simulink model "NHR9410Model24k_2020b"  (R2020b)
settings: Solver=VariableStepAuto  StartTime=0.0  StopTime=1  FixedStep=0.001  RelTol=1e-3
libraries: simulink x85, fl_lib x46, powerlib_meascontrol x27, simulink_extras x24, nesl_utility x13, fl_ps_legacy_lib x3
(part 3 of 4)

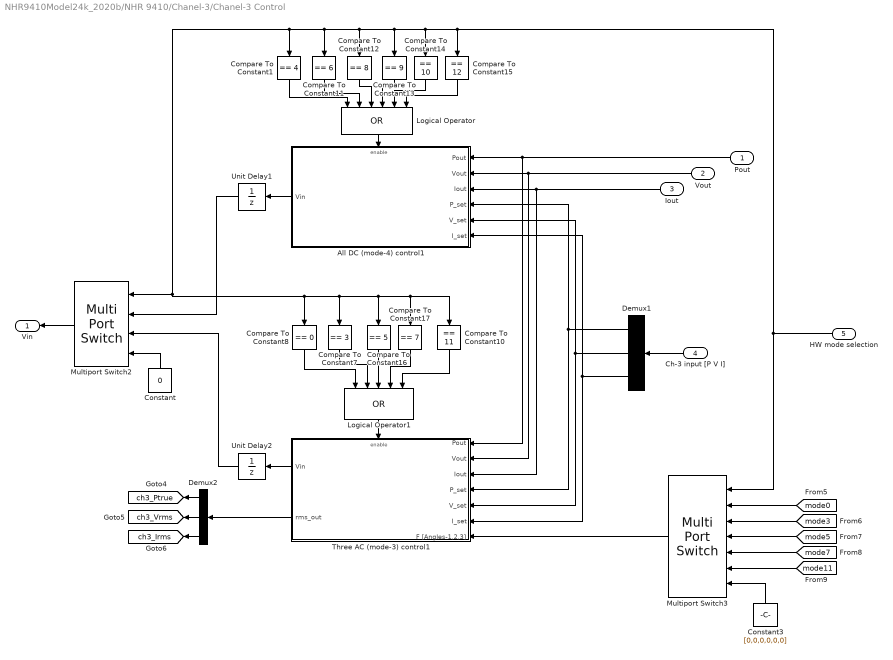
== system NHR9410Model24k_2020b/NHR 9410/Chanel-3/Chanel-3 Control ==
  Pout : Inport
  Vout : Inport  Port=2
  Iout : Inport  Port=3
  Ch-3 input [P V I] : Inport  Port=4
  HW mode selection : Inport  Port=5
  All DC (mode-4) control1 : Subsystem
      settings: MinAlgLoopOccurrences=on
  Compare To Constant1 : simulink/Logic and Bit Operations/Compare To Constant  relop===  const=4  OutDataTypeStr=boolean
  Compare To Constant10 : simulink/Logic and Bit Operations/Compare To Constant  relop===  const=11  OutDataTypeStr=boolean
  Compare To Constant11 : simulink/Logic and Bit Operations/Compare To Constant  relop===  const=6  OutDataTypeStr=boolean
  Compare To Constant12 : simulink/Logic and Bit Operations/Compare To Constant  relop===  const=8  OutDataTypeStr=boolean
  Compare To Constant13 : simulink/Logic and Bit Operations/Compare To Constant  relop===  const=9  OutDataTypeStr=boolean
  Compare To Constant14 : simulink/Logic and Bit Operations/Compare To Constant  relop===  const=10  OutDataTypeStr=boolean
  Compare To Constant15 : simulink/Logic and Bit Operations/Compare To Constant  relop===  const=12  OutDataTypeStr=boolean
  Compare To Constant16 : simulink/Logic and Bit Operations/Compare To Constant  relop===  const=5  OutDataTypeStr=boolean
  Compare To Constant17 : simulink/Logic and Bit Operations/Compare To Constant  relop===  const=7  OutDataTypeStr=boolean
  Compare To Constant7 : simulink/Logic and Bit Operations/Compare To Constant  relop===  const=3  OutDataTypeStr=boolean
  Compare To Constant8 : simulink/Logic and Bit Operations/Compare To Constant  relop===  const=0  OutDataTypeStr=boolean
  Constant : Constant  Value=0
  Constant3 : Constant  Value=[0,0,0,0,0,0]
  Demux1 : Demux  Outputs=3
  Demux2 : Demux  Outputs=3
  Logical Operator : Logic  Operator=OR  Inputs=6  AllPortsSameDT=off  OutDataTypeStr=boolean
  Logical Operator1 : Logic  Operator=OR  Inputs=5  AllPortsSameDT=off  OutDataTypeStr=boolean
  Multiport Switch2 : MultiPortSwitch  DataPortOrder=Specify indices  Inputs=13  DataPortIndices={[4,6,8,9,10,12],[0,3,5,7,11]}  DataPortForDefault=Additional data port  DiagnosticForDefault=None
  Multiport Switch3 : MultiPortSwitch  DataPortOrder=Specify indices  Inputs=13  DataPortIndices={0,3,5,7,11}  DataPortForDefault=Additional data port  DiagnosticForDefault=None
  Three AC (mode-3) control1 : Subsystem
      settings: MinAlgLoopOccurrences=on
  Unit Delay1 : UnitDelay  SampleTime=-1  HasFrameUpgradeWarning=on
  Unit Delay2 : UnitDelay  SampleTime=-1  HasFrameUpgradeWarning=on
  Vin : Outport  VectorParamsAs1DForOutWhenUnconnected=off
  tag scope: ch3_Irms=global, ch3_Ptrue=global, ch3_Vrms=global
  wires:
  Demux2/2 -> [ch3_Vrms]
  Demux2/3 -> [ch3_Irms]
  Demux2/1 -> [ch3_Ptrue]
  Multiport Switch3/1 -> Three AC (mode-3) control1/7(F [Angles-1,2,3])
  Compare To Constant17/1 -> Logical Operator1/4
  Iout/1 -> All DC (mode-4) control1/3(Iout), Three AC (mode-3) control1/3(Iout)
  Three AC (mode-3) control1/1(Vin) -> Unit Delay2/1
  Multiport Switch2/1 -> Vin/1
  [mode11] -> Multiport Switch3/6
  Logical Operator1/1 -> Three AC (mode-3) control1/Enable
  Demux1/1 -> All DC (mode-4) control1/4(P_set), Three AC (mode-3) control1/4(P_set)
  Compare To Constant10/1 -> Logical Operator1/5
  [mode0] -> Multiport Switch3/2
  Compare To Constant8/1 -> Logical Operator1/1
  Demux1/2 -> All DC (mode-4) control1/5(V_set), Three AC (mode-3) control1/5(V_set)
  Pout/1 -> All DC (mode-4) control1/1(Pout), Three AC (mode-3) control1/1(Pout)
  Demux1/3 -> All DC (mode-4) control1/6(I_set), Three AC (mode-3) control1/6(I_set)
  Vout/1 -> All DC (mode-4) control1/2(Vout), Three AC (mode-3) control1/2(Vout)
  [mode5] -> Multiport Switch3/4
  Ch-3 input [P V I]/1 -> Demux1/1
  [mode3] -> Multiport Switch3/3
  [mode7] -> Multiport Switch3/5
  Compare To Constant16/1 -> Logical Operator1/3
  All DC (mode-4) control1/1(Vin) -> Unit Delay1/1
  Constant3/1 -> Multiport Switch3/7
  Compare To Constant7/1 -> Logical Operator1/2
  Constant/1 -> Multiport Switch2/4
  Three AC (mode-3) control1/2(rms_out) -> Demux2/1
  Logical Operator/1 -> All DC (mode-4) control1/Enable
  Compare To Constant15/1 -> Logical Operator/6
  Compare To Constant14/1 -> Logical Operator/5
  Compare To Constant13/1 -> Logical Operator/4
  Compare To Constant1/1 -> Logical Operator/1
  Compare To Constant11/1 -> Logical Operator/2
  HW mode selection/1 -> Compare To Constant8/1, Compare To Constant10/1, Compare To Constant17/1, Compare To Constant16/1, Compare To Constant7/1, Multiport Switch2/1, Compare To Constant1/1, Compare To Constant11/1, Compare To Constant12/1, Compare To Constant13/1, Compare To Constant14/1, Compare To Constant15/1, Multiport Switch3/1
  Compare To Constant12/1 -> Logical Operator/3
  Unit Delay1/1 -> Multiport Switch2/2
  Unit Delay2/1 -> Multiport Switch2/3

== system NHR9410Model24k_2020b/NHR 9410 Safety Settings/Safety Ch-1/Trip signal generator (max) Sink Current ==
  signal_in : Inport
  Constant : Constant  Value=Simaxsnk1  VectorParams1D=off
  Constant1 : Constant  Value=0
  Relational Operator : RelationalOperator  OutDataTypeStr=boolean  RndMeth=Simplest
  trip signal gen : Subsystem
  signal_trip : Outport  VectorParamsAs1DForOutWhenUnconnected=off
  wires:
  signal_in/1 -> trip signal gen/1(signal in)
  trip signal gen/1(trip_out) -> signal_trip/1
  Constant/1 -> Relational Operator/1
  Constant1/1 -> Relational Operator/2
  Relational Operator/1 -> trip signal gen/Enable

== system NHR9410Model24k_2020b/NHR 9410 Safety Settings/Safety Ch-1/Trip signal generator (max) Sink Power ==
  signal_in : Inport
  Constant : Constant  Value=Spmaxsnk1  VectorParams1D=off
  Constant1 : Constant  Value=0
  Relational Operator : RelationalOperator  OutDataTypeStr=boolean  RndMeth=Simplest
  trip signal gen : Subsystem
  signal_trip : Outport  VectorParamsAs1DForOutWhenUnconnected=off
  wires:
  Relational Operator/1 -> trip signal gen/Enable
  Constant1/1 -> Relational Operator/2
  Constant/1 -> Relational Operator/1
  trip signal gen/1(trip_out) -> signal_trip/1
  signal_in/1 -> trip signal gen/1(signal in)

== system NHR9410Model24k_2020b/NHR 9410 Safety Settings/Safety Ch-1/Trip signal generator (max) Source Current ==
  signal_in : Inport
  Constant : Constant  Value=Simaxsrc1  VectorParams1D=off
  Constant1 : Constant  Value=0
  Relational Operator : RelationalOperator  OutDataTypeStr=boolean  RndMeth=Simplest
  trip signal gen : Subsystem
  signal_trip : Outport  VectorParamsAs1DForOutWhenUnconnected=off
  wires:
  Relational Operator/1 -> trip signal gen/Enable
  Constant1/1 -> Relational Operator/2
  Constant/1 -> Relational Operator/1
  trip signal gen/1(trip_out) -> signal_trip/1
  signal_in/1 -> trip signal gen/1(signal in)

== system NHR9410Model24k_2020b/NHR 9410 Safety Settings/Safety Ch-1/Trip signal generator (max) Source Power ==
  signal_in : Inport
  Constant : Constant  Value=Spmaxsrc1  VectorParams1D=off
  Constant1 : Constant  Value=0
  Relational Operator : RelationalOperator  OutDataTypeStr=boolean  RndMeth=Simplest
  trip signal gen : Subsystem
  signal_trip : Outport  VectorParamsAs1DForOutWhenUnconnected=off
  wires:
  signal_in/1 -> trip signal gen/1(signal in)
  trip signal gen/1(trip_out) -> signal_trip/1
  Constant/1 -> Relational Operator/1
  Constant1/1 -> Relational Operator/2
  Relational Operator/1 -> trip signal gen/Enable

== system NHR9410Model24k_2020b/NHR 9410 Safety Settings/Safety Ch-1/Trip signal generator (max) Voltage ==
  signal_in : Inport
  Constant : Constant  Value=Svmax1  VectorParams1D=off
  Constant1 : Constant  Value=0
  Relational Operator : RelationalOperator  OutDataTypeStr=boolean  RndMeth=Simplest
  trip signal gen : Subsystem
  signal_trip : Outport  VectorParamsAs1DForOutWhenUnconnected=off
  wires:
  signal_in/1 -> trip signal gen/1(signal in)
  trip signal gen/1(trip_out) -> signal_trip/1
  Constant/1 -> Relational Operator/1
  Constant1/1 -> Relational Operator/2
  Relational Operator/1 -> trip signal gen/Enable

== system NHR9410Model24k_2020b/NHR 9410 Safety Settings/Safety Ch-1/Trip signal generator (min) Voltage ==
  signal_in : Inport
  Constant : Constant  Value=Svmin1  VectorParams1D=off
  Constant1 : Constant  Value=0
  Relational Operator : RelationalOperator  OutDataTypeStr=boolean  RndMeth=Simplest
  trip signal gen : Subsystem
  signal_trip : Outport  VectorParamsAs1DForOutWhenUnconnected=off
  wires:
  Relational Operator/1 -> trip signal gen/Enable
  Constant1/1 -> Relational Operator/2
  Constant/1 -> Relational Operator/1
  trip signal gen/1(trip_out) -> signal_trip/1
  signal_in/1 -> trip signal gen/1(signal in)

== system NHR9410Model24k_2020b/NHR 9410 Safety Settings/Safety Ch-1/Trip signal generator (peak) Current ==
  signal_in : Inport
  peak_ctrl : Inport  Port=2
  Constant : Constant  Value=Ipeaken1  VectorParams1D=off
  Constant1 : Constant
  Logical Operator : Logic  AllPortsSameDT=off  OutDataTypeStr=boolean
  Relational Operator : RelationalOperator  Operator===  OutDataTypeStr=boolean  RndMeth=Simplest
  trip signal gen : Subsystem
  signal_trip : Outport  VectorParamsAs1DForOutWhenUnconnected=off
  wires:
  Constant1/1 -> Relational Operator/2
  Constant/1 -> Relational Operator/1
  signal_in/1 -> trip signal gen/1(signal in)
  trip signal gen/1(trip_out) -> signal_trip/1
  Relational Operator/1 -> Logical Operator/1
  Logical Operator/1 -> trip signal gen/Enable
  peak_ctrl/1 -> Logical Operator/2

== system NHR9410Model24k_2020b/NHR 9410 Safety Settings/Safety Ch-1/Trip signal generator (peak) Voltage ==
  signal_in : Inport
  peak_ctrl : Inport  Port=2
  Constant : Constant  Value=Vpeaken1  VectorParams1D=off
  Constant1 : Constant
  Logical Operator : Logic  AllPortsSameDT=off  OutDataTypeStr=boolean
  Relational Operator : RelationalOperator  Operator===  OutDataTypeStr=boolean  RndMeth=Simplest
  trip signal gen : Subsystem
  signal_trip : Outport  VectorParamsAs1DForOutWhenUnconnected=off
  wires:
  signal_in/1 -> trip signal gen/1(signal in)
  trip signal gen/1(trip_out) -> signal_trip/1
  Constant/1 -> Relational Operator/1
  Constant1/1 -> Relational Operator/2
  Relational Operator/1 -> Logical Operator/1
  Logical Operator/1 -> trip signal gen/Enable
  peak_ctrl/1 -> Logical Operator/2

== system NHR9410Model24k_2020b/NHR 9410 Safety Settings/Safety Ch-2/Trip signal generator (max) Sink Current ==
  signal_in : Inport
  Constant : Constant  Value=Simaxsnk2  VectorParams1D=off
  Constant1 : Constant  Value=0
  Relational Operator : RelationalOperator  OutDataTypeStr=boolean  RndMeth=Simplest
  trip signal gen : Subsystem
  signal_trip : Outport  VectorParamsAs1DForOutWhenUnconnected=off
  wires:
  Relational Operator/1 -> trip signal gen/Enable
  Constant1/1 -> Relational Operator/2
  Constant/1 -> Relational Operator/1
  trip signal gen/1(trip_out) -> signal_trip/1
  signal_in/1 -> trip signal gen/1(signal in)

== system NHR9410Model24k_2020b/NHR 9410 Safety Settings/Safety Ch-2/Trip signal generator (max) Sink Power ==
  signal_in : Inport
  Constant : Constant  Value=Spmaxsnk2  VectorParams1D=off
  Constant1 : Constant  Value=0
  Relational Operator : RelationalOperator  OutDataTypeStr=boolean  RndMeth=Simplest
  trip signal gen : Subsystem
  signal_trip : Outport  VectorParamsAs1DForOutWhenUnconnected=off
  wires:
  signal_in/1 -> trip signal gen/1(signal in)
  trip signal gen/1(trip_out) -> signal_trip/1
  Constant/1 -> Relational Operator/1
  Constant1/1 -> Relational Operator/2
  Relational Operator/1 -> trip signal gen/Enable

== system NHR9410Model24k_2020b/NHR 9410 Safety Settings/Safety Ch-2/Trip signal generator (max) Source Current ==
  signal_in : Inport
  Constant : Constant  Value=Simaxsrc2  VectorParams1D=off
  Constant1 : Constant  Value=0
  Relational Operator : RelationalOperator  OutDataTypeStr=boolean  RndMeth=Simplest
  trip signal gen : Subsystem
  signal_trip : Outport  VectorParamsAs1DForOutWhenUnconnected=off
  wires:
  signal_in/1 -> trip signal gen/1(signal in)
  trip signal gen/1(trip_out) -> signal_trip/1
  Constant/1 -> Relational Operator/1
  Constant1/1 -> Relational Operator/2
  Relational Operator/1 -> trip signal gen/Enable

== system NHR9410Model24k_2020b/NHR 9410 Safety Settings/Safety Ch-2/Trip signal generator (max) Source Power ==
  signal_in : Inport
  Constant : Constant  Value=Spmaxsrc2  VectorParams1D=off
  Constant1 : Constant  Value=0
  Relational Operator : RelationalOperator  OutDataTypeStr=boolean  RndMeth=Simplest
  trip signal gen : Subsystem
  signal_trip : Outport  VectorParamsAs1DForOutWhenUnconnected=off
  wires:
  Relational Operator/1 -> trip signal gen/Enable
  Constant1/1 -> Relational Operator/2
  Constant/1 -> Relational Operator/1
  trip signal gen/1(trip_out) -> signal_trip/1
  signal_in/1 -> trip signal gen/1(signal in)

== system NHR9410Model24k_2020b/NHR 9410 Safety Settings/Safety Ch-2/Trip signal generator (max) Voltage ==
  signal_in : Inport
  Constant : Constant  Value=Svmax2  VectorParams1D=off
  Constant1 : Constant  Value=0
  Relational Operator : RelationalOperator  OutDataTypeStr=boolean  RndMeth=Simplest
  trip signal gen : Subsystem
  signal_trip : Outport  VectorParamsAs1DForOutWhenUnconnected=off
  wires:
  Relational Operator/1 -> trip signal gen/Enable
  Constant1/1 -> Relational Operator/2
  Constant/1 -> Relational Operator/1
  trip signal gen/1(trip_out) -> signal_trip/1
  signal_in/1 -> trip signal gen/1(signal in)

== system NHR9410Model24k_2020b/NHR 9410 Safety Settings/Safety Ch-2/Trip signal generator (min) Voltage ==
  signal_in : Inport
  Constant : Constant  Value=Svmin2  VectorParams1D=off
  Constant1 : Constant  Value=0
  Relational Operator : RelationalOperator  OutDataTypeStr=boolean  RndMeth=Simplest
  trip signal gen : Subsystem
  signal_trip : Outport  VectorParamsAs1DForOutWhenUnconnected=off
  wires:
  signal_in/1 -> trip signal gen/1(signal in)
  trip signal gen/1(trip_out) -> signal_trip/1
  Constant/1 -> Relational Operator/1
  Constant1/1 -> Relational Operator/2
  Relational Operator/1 -> trip signal gen/Enable

== system NHR9410Model24k_2020b/NHR 9410 Safety Settings/Safety Ch-2/Trip signal generator (peak) Current ==
  signal_in : Inport
  peak_ctrl : Inport  Port=2
  Constant : Constant  Value=Ipeaken2  VectorParams1D=off
  Constant1 : Constant
  Logical Operator : Logic  AllPortsSameDT=off  OutDataTypeStr=boolean
  Relational Operator : RelationalOperator  Operator===  OutDataTypeStr=boolean  RndMeth=Simplest
  trip signal gen : Subsystem
  signal_trip : Outport  VectorParamsAs1DForOutWhenUnconnected=off
  wires:
  signal_in/1 -> trip signal gen/1(signal in)
  trip signal gen/1(trip_out) -> signal_trip/1
  Constant/1 -> Relational Operator/1
  Constant1/1 -> Relational Operator/2
  peak_ctrl/1 -> Logical Operator/2
  Relational Operator/1 -> Logical Operator/1
  Logical Operator/1 -> trip signal gen/Enable

== system NHR9410Model24k_2020b/NHR 9410 Safety Settings/Safety Ch-2/Trip signal generator (peak) Voltage ==
  signal_in : Inport
  peak_ctrl : Inport  Port=2
  Constant : Constant  Value=Vpeaken2  VectorParams1D=off
  Constant1 : Constant
  Logical Operator : Logic  AllPortsSameDT=off  OutDataTypeStr=boolean
  Relational Operator : RelationalOperator  Operator===  OutDataTypeStr=boolean  RndMeth=Simplest
  trip signal gen : Subsystem
  signal_trip : Outport  VectorParamsAs1DForOutWhenUnconnected=off
  wires:
  Constant1/1 -> Relational Operator/2
  Constant/1 -> Relational Operator/1
  trip signal gen/1(trip_out) -> signal_trip/1
  signal_in/1 -> trip signal gen/1(signal in)
  peak_ctrl/1 -> Logical Operator/2
  Logical Operator/1 -> trip signal gen/Enable
  Relational Operator/1 -> Logical Operator/1

== system NHR9410Model24k_2020b/NHR 9410 Safety Settings/Safety Ch-3/Trip signal generator (max) Sink Current ==
  signal_in : Inport
  Constant : Constant  Value=Simaxsnk3  VectorParams1D=off
  Constant1 : Constant  Value=0
  Relational Operator : RelationalOperator  OutDataTypeStr=boolean  RndMeth=Simplest
  trip signal gen : Subsystem
  signal_trip : Outport  VectorParamsAs1DForOutWhenUnconnected=off
  wires:
  signal_in/1 -> trip signal gen/1(signal in)
  trip signal gen/1(trip_out) -> signal_trip/1
  Constant/1 -> Relational Operator/1
  Constant1/1 -> Relational Operator/2
  Relational Operator/1 -> trip signal gen/Enable

== system NHR9410Model24k_2020b/NHR 9410 Safety Settings/Safety Ch-3/Trip signal generator (max) Sink Power ==
  signal_in : Inport
  Constant : Constant  Value=Spmaxsnk3  VectorParams1D=off
  Constant1 : Constant  Value=0
  Relational Operator : RelationalOperator  OutDataTypeStr=boolean  RndMeth=Simplest
  trip signal gen : Subsystem
  signal_trip : Outport  VectorParamsAs1DForOutWhenUnconnected=off
  wires:
  Relational Operator/1 -> trip signal gen/Enable
  Constant1/1 -> Relational Operator/2
  Constant/1 -> Relational Operator/1
  trip signal gen/1(trip_out) -> signal_trip/1
  signal_in/1 -> trip signal gen/1(signal in)

== system NHR9410Model24k_2020b/NHR 9410 Safety Settings/Safety Ch-3/Trip signal generator (max) Source Current ==
  signal_in : Inport
  Constant : Constant  Value=Simaxsrc3  VectorParams1D=off
  Constant1 : Constant  Value=0
  Relational Operator : RelationalOperator  OutDataTypeStr=boolean  RndMeth=Simplest
  trip signal gen : Subsystem
  signal_trip : Outport  VectorParamsAs1DForOutWhenUnconnected=off
  wires:
  Relational Operator/1 -> trip signal gen/Enable
  Constant1/1 -> Relational Operator/2
  Constant/1 -> Relational Operator/1
  trip signal gen/1(trip_out) -> signal_trip/1
  signal_in/1 -> trip signal gen/1(signal in)

== system NHR9410Model24k_2020b/NHR 9410 Safety Settings/Safety Ch-3/Trip signal generator (max) Source Power ==
  signal_in : Inport
  Constant : Constant  Value=Spmaxsrc3  VectorParams1D=off
  Constant1 : Constant  Value=0
  Relational Operator : RelationalOperator  OutDataTypeStr=boolean  RndMeth=Simplest
  trip signal gen : Subsystem
  signal_trip : Outport  VectorParamsAs1DForOutWhenUnconnected=off
  wires:
  signal_in/1 -> trip signal gen/1(signal in)
  trip signal gen/1(trip_out) -> signal_trip/1
  Constant/1 -> Relational Operator/1
  Constant1/1 -> Relational Operator/2
  Relational Operator/1 -> trip signal gen/Enable

== system NHR9410Model24k_2020b/NHR 9410 Safety Settings/Safety Ch-3/Trip signal generator (max) Voltage ==
  signal_in : Inport
  Constant : Constant  Value=Svmax3  VectorParams1D=off
  Constant1 : Constant  Value=0
  Relational Operator : RelationalOperator  OutDataTypeStr=boolean  RndMeth=Simplest
  trip signal gen : Subsystem
  signal_trip : Outport  VectorParamsAs1DForOutWhenUnconnected=off
  wires:
  signal_in/1 -> trip signal gen/1(signal in)
  trip signal gen/1(trip_out) -> signal_trip/1
  Constant/1 -> Relational Operator/1
  Constant1/1 -> Relational Operator/2
  Relational Operator/1 -> trip signal gen/Enable

== system NHR9410Model24k_2020b/NHR 9410 Safety Settings/Safety Ch-3/Trip signal generator (min) Voltage ==
  signal_in : Inport
  Constant : Constant  Value=Svmin3  VectorParams1D=off
  Constant1 : Constant  Value=0
  Relational Operator : RelationalOperator  OutDataTypeStr=boolean  RndMeth=Simplest
  trip signal gen : Subsystem
  signal_trip : Outport  VectorParamsAs1DForOutWhenUnconnected=off
  wires:
  Relational Operator/1 -> trip signal gen/Enable
  Constant1/1 -> Relational Operator/2
  Constant/1 -> Relational Operator/1
  trip signal gen/1(trip_out) -> signal_trip/1
  signal_in/1 -> trip signal gen/1(signal in)

== system NHR9410Model24k_2020b/NHR 9410 Safety Settings/Safety Ch-3/Trip signal generator (peak) Current ==
  signal_in : Inport
  peak_ctrl : Inport  Port=2
  Constant : Constant  Value=Ipeaken3  VectorParams1D=off
  Constant1 : Constant
  Logical Operator : Logic  AllPortsSameDT=off  OutDataTypeStr=boolean
  Relational Operator : RelationalOperator  Operator===  OutDataTypeStr=boolean  RndMeth=Simplest
  trip signal gen : Subsystem
  signal_trip : Outport  VectorParamsAs1DForOutWhenUnconnected=off
  wires:
  Constant1/1 -> Relational Operator/2
  Constant/1 -> Relational Operator/1
  trip signal gen/1(trip_out) -> signal_trip/1
  signal_in/1 -> trip signal gen/1(signal in)
  peak_ctrl/1 -> Logical Operator/2
  Logical Operator/1 -> trip signal gen/Enable
  Relational Operator/1 -> Logical Operator/1

== system NHR9410Model24k_2020b/NHR 9410 Safety Settings/Safety Ch-3/Trip signal generator (peak) Voltage ==
  signal_in : Inport
  peak_ctrl : Inport  Port=2
  Constant : Constant  Value=Vpeaken3  VectorParams1D=off
  Constant1 : Constant
  Logical Operator : Logic  AllPortsSameDT=off  OutDataTypeStr=boolean
  Relational Operator : RelationalOperator  Operator===  OutDataTypeStr=boolean  RndMeth=Simplest
  trip signal gen : Subsystem
  signal_trip : Outport  VectorParamsAs1DForOutWhenUnconnected=off
  wires:
  signal_in/1 -> trip signal gen/1(signal in)
  trip signal gen/1(trip_out) -> signal_trip/1
  Constant/1 -> Relational Operator/1
  Constant1/1 -> Relational Operator/2
  peak_ctrl/1 -> Logical Operator/2
  Logical Operator/1 -> trip signal gen/Enable
  Relational Operator/1 -> Logical Operator/1

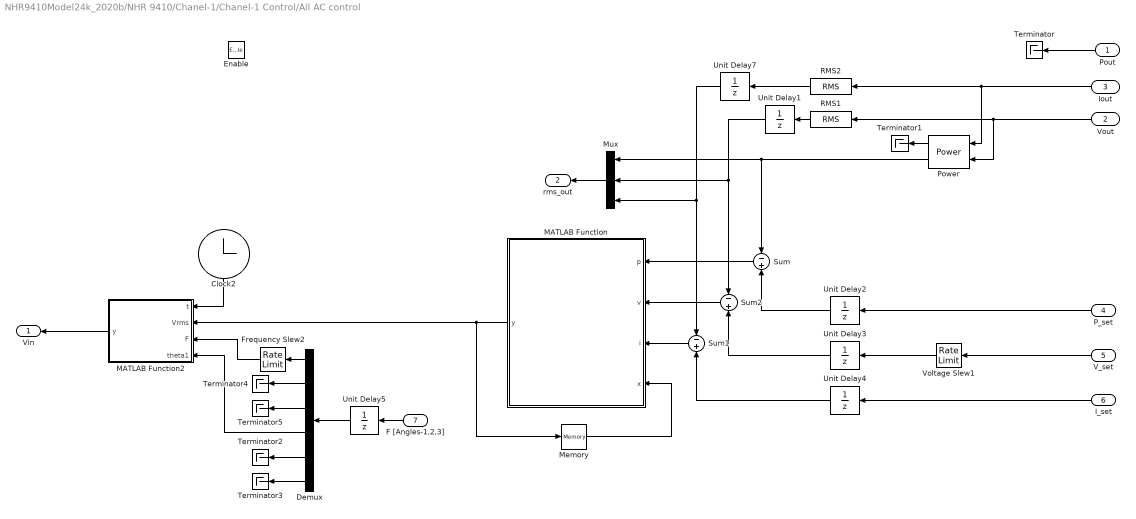
== system NHR9410Model24k_2020b/NHR 9410/Chanel-1/Chanel-1 Control/All AC control ==
  Pout : Inport
  Vout : Inport  Port=2
  Iout : Inport  Port=3
  P_set : Inport  Port=4
  V_set : Inport  Port=5
  I_set : Inport  Port=6
  F [Angles-1,2,3] : Inport  Port=7
  Enable : EnablePort
  Clock2 : Clock
  Demux : Demux  Outputs=6
  Frequency Slew2 : RateLimiter  RisingSlewLimit=FslewAC  FallingSlewLimit=-FslewAC  SampleTimeMode=inherited  LinearizeAsGain=off
  MATLAB Function : MATLAB Function  TreatAsAtomicUnit=on
  MATLAB Function2 : MATLAB Function  TreatAsAtomicUnit=on
  Memory : Memory
  Mux : Mux  Inputs=3
  Power : powerlib_meascontrol/Measurements/Power  Freq=60  Vinit=[0, 0]  Iinit=[0, 0]  Ts=0
  RMS1 : powerlib_meascontrol/Measurements/RMS  TrueRMS=on  Freq=60  RMSInit=0  Ts=0
  RMS2 : powerlib_meascontrol/Measurements/RMS  TrueRMS=on  Freq=60  RMSInit=0  Ts=0
  Sum : Sum  Inputs=-+
  Sum1 : Sum  Inputs=-+
  Sum2 : Sum  Inputs=-+
  Terminator{,1..5} (6 alike) : Terminator
  Unit Delay{1..5,7} (6 alike) : UnitDelay  SampleTime=-1  HasFrameUpgradeWarning=on
  Voltage Slew1 : RateLimiter  RisingSlewLimit=VslewAC  FallingSlewLimit=-VslewAC  SampleTimeMode=inherited  LinearizeAsGain=off
  Vin : Outport  VectorParamsAs1DForOutWhenUnconnected=off
  rms_out : Outport  Port=2  VectorParamsAs1DForOutWhenUnconnected=off
  wires:
  Voltage Slew1/1 -> Unit Delay3/1
  Frequency Slew2/1 -> MATLAB Function2/3(F)
  V_set/1 -> Voltage Slew1/1
  F [Angles-1,2,3]/1 -> Unit Delay5/1
  Demux/6 -> Terminator3/1
  Demux/3 -> Terminator5/1
  Mux/1 -> rms_out/1
  Power/1 -> Sum/1, Mux/1
  MATLAB Function2/1(y) -> Vin/1
  Clock2/1 -> MATLAB Function2/1(t)
  Memory/1 -> MATLAB Function/4(x)
  RMS2/1 -> Unit Delay7/1
  RMS1/1 -> Unit Delay1/1
  P_set/1 -> Unit Delay2/1
  I_set/1 -> Unit Delay4/1
  Sum1/1 -> MATLAB Function/3(i)
  Sum2/1 -> MATLAB Function/2(v)
  Sum/1 -> MATLAB Function/1(p)
  Power/2 -> Terminator1/1
  Pout/1 -> Terminator/1
  Iout/1 -> Power/2, RMS2/1
  MATLAB Function/1(y) -> Memory/1, MATLAB Function2/2(Vrms)
  Vout/1 -> Power/1, RMS1/1
  Demux/1 -> Frequency Slew2/1
  Demux/2 -> Terminator4/1
  Demux/5 -> Terminator2/1
  Demux/4 -> MATLAB Function2/4(theta1)
  Unit Delay7/1 -> Sum1/1, Mux/3
  Unit Delay1/1 -> Sum2/1, Mux/2
  Unit Delay2/1 -> Sum/2
  Unit Delay3/1 -> Sum2/2
  Unit Delay4/1 -> Sum1/2
  Unit Delay5/1 -> Demux/1

== system NHR9410Model24k_2020b/NHR 9410/Chanel-1/Chanel-1 Control/All DC control ==
  Pout : Inport
  Vout : Inport  Port=2
  Iout : Inport  Port=3
  P_set : Inport  Port=4
  V_set : Inport  Port=5
  I_set : Inport  Port=6
  Enable : EnablePort
  Current Slew : RateLimiter  RisingSlewLimit=IslewDC  FallingSlewLimit=-IslewDC  SampleTimeMode=inherited  LinearizeAsGain=off
  MATLAB Function : MATLAB Function  TreatAsAtomicUnit=on
  Memory : Memory
  Power Slew : RateLimiter  RisingSlewLimit=PslewDC  FallingSlewLimit=-PslewDC  SampleTimeMode=inherited  LinearizeAsGain=off
  Sum : Sum  Inputs=-+
  Sum1 : Sum  Inputs=-+
  Sum2 : Sum  Inputs=-+
  Unit Delay{,1..5} (6 alike) : UnitDelay  SampleTime=-1  HasFrameUpgradeWarning=on
  Voltage Slew : RateLimiter  RisingSlewLimit=VslewDC  FallingSlewLimit=-VslewDC  SampleTimeMode=inherited  LinearizeAsGain=off
  Vin : Outport  VectorParamsAs1DForOutWhenUnconnected=off
  wires:
  Power Slew/1 -> Unit Delay4/1
  Voltage Slew/1 -> Unit Delay3/1
  Current Slew/1 -> Unit Delay5/1
  I_set/1 -> Current Slew/1
  V_set/1 -> Voltage Slew/1
  P_set/1 -> Power Slew/1
  MATLAB Function/1(y) -> Memory/1, Vin/1
  Iout/1 -> Unit Delay/1
  Pout/1 -> Unit Delay2/1
  Sum/1 -> MATLAB Function/1(p)
  Sum1/1 -> MATLAB Function/3(i)
  Sum2/1 -> MATLAB Function/2(v)
  Memory/1 -> MATLAB Function/4(x)
  Unit Delay2/1 -> Sum/1
  Vout/1 -> Unit Delay1/1
  Unit Delay/1 -> Sum1/1
  Unit Delay1/1 -> Sum2/1
  Unit Delay4/1 -> Sum/2
  Unit Delay3/1 -> Sum2/2
  Unit Delay5/1 -> Sum1/2

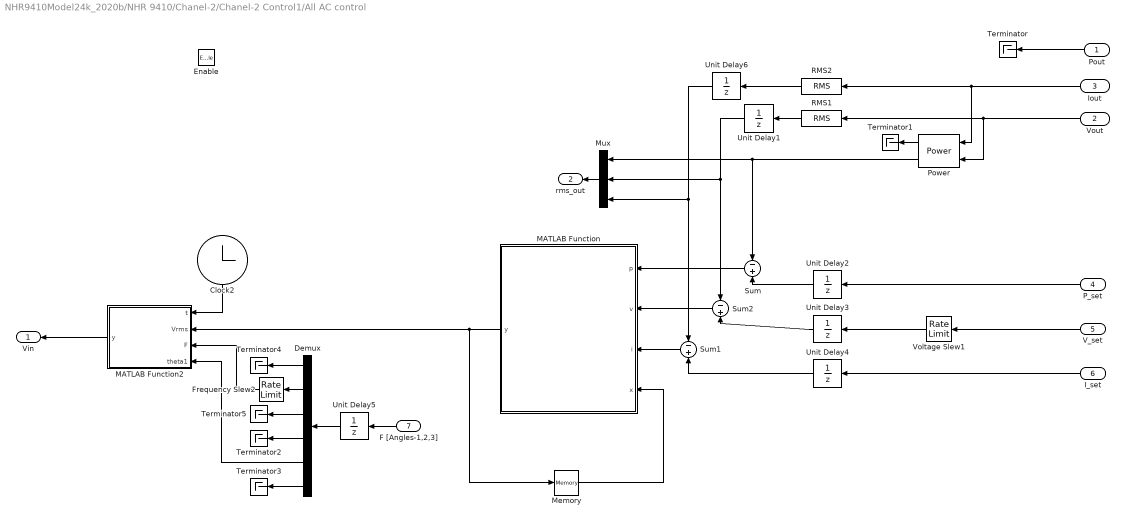
== system NHR9410Model24k_2020b/NHR 9410/Chanel-2/Chanel-2 Control1/All AC control ==
  Pout : Inport
  Vout : Inport  Port=2
  Iout : Inport  Port=3
  P_set : Inport  Port=4
  V_set : Inport  Port=5
  I_set : Inport  Port=6
  F [Angles-1,2,3] : Inport  Port=7
  Enable : EnablePort
  Clock2 : Clock
  Demux : Demux  Outputs=6
  Frequency Slew2 : RateLimiter  RisingSlewLimit=FslewAC  FallingSlewLimit=-FslewAC  SampleTimeMode=inherited  LinearizeAsGain=off
  MATLAB Function : MATLAB Function  TreatAsAtomicUnit=on
  MATLAB Function2 : MATLAB Function  TreatAsAtomicUnit=on
  Memory : Memory
  Mux : Mux  Inputs=3
  Power : powerlib_meascontrol/Measurements/Power  Freq=60  Vinit=[0, 0]  Iinit=[0, 0]  Ts=0
  RMS1 : powerlib_meascontrol/Measurements/RMS  TrueRMS=on  Freq=60  RMSInit=0  Ts=0
  RMS2 : powerlib_meascontrol/Measurements/RMS  TrueRMS=on  Freq=60  RMSInit=0  Ts=0
  Sum : Sum  Inputs=-+
  Sum1 : Sum  Inputs=-+
  Sum2 : Sum  Inputs=-+
  Terminator{,1..5} (6 alike) : Terminator
  Unit Delay{1..6} (6 alike) : UnitDelay  SampleTime=-1  HasFrameUpgradeWarning=on
  Voltage Slew1 : RateLimiter  RisingSlewLimit=VslewAC  FallingSlewLimit=-VslewAC  SampleTimeMode=inherited  LinearizeAsGain=off
  Vin : Outport  VectorParamsAs1DForOutWhenUnconnected=off
  rms_out : Outport  Port=2  VectorParamsAs1DForOutWhenUnconnected=off
  wires:
  Vout/1 -> RMS1/1, Power/1
  MATLAB Function/1(y) -> MATLAB Function2/2(Vrms), Memory/1
  Iout/1 -> RMS2/1, Power/2
  Pout/1 -> Terminator/1
  Power/2 -> Terminator1/1
  Sum/1 -> MATLAB Function/1(p)
  Sum2/1 -> MATLAB Function/2(v)
  Sum1/1 -> MATLAB Function/3(i)
  I_set/1 -> Unit Delay4/1
  P_set/1 -> Unit Delay2/1
  RMS1/1 -> Unit Delay1/1
  RMS2/1 -> Unit Delay6/1
  Memory/1 -> MATLAB Function/4(x)
  Clock2/1 -> MATLAB Function2/1(t)
  MATLAB Function2/1(y) -> Vin/1
  Power/1 -> Sum/1, Mux/1
  Mux/1 -> rms_out/1
  Demux/3 -> Terminator5/1
  Demux/6 -> Terminator3/1
  F [Angles-1,2,3]/1 -> Unit Delay5/1
  Demux/1 -> Terminator4/1
  Demux/4 -> Terminator2/1
  Demux/5 -> MATLAB Function2/4(theta1)
  V_set/1 -> Voltage Slew1/1
  Demux/2 -> Frequency Slew2/1
  Frequency Slew2/1 -> MATLAB Function2/3(F)
  Voltage Slew1/1 -> Unit Delay3/1
  Unit Delay6/1 -> Sum1/1, Mux/3
  Unit Delay1/1 -> Sum2/1, Mux/2
  Unit Delay2/1 -> Sum/2
  Unit Delay3/1 -> Sum2/2
  Unit Delay4/1 -> Sum1/2
  Unit Delay5/1 -> Demux/1

== system NHR9410Model24k_2020b/NHR 9410/Chanel-2/Chanel-2 Control1/All DC control ==
  Pout : Inport
  Vout : Inport  Port=2
  Iout : Inport  Port=3
  P_set : Inport  Port=4
  V_set : Inport  Port=5
  I_set : Inport  Port=6
  Enable : EnablePort
  Current Slew : RateLimiter  RisingSlewLimit=IslewDC  FallingSlewLimit=-IslewDC  SampleTimeMode=inherited  LinearizeAsGain=off
  MATLAB Function : MATLAB Function  TreatAsAtomicUnit=on
  Memory : Memory
  Power Slew : RateLimiter  RisingSlewLimit=PslewDC  FallingSlewLimit=-PslewDC  SampleTimeMode=inherited  LinearizeAsGain=off
  Sum : Sum  Inputs=-+
  Sum1 : Sum  Inputs=-+
  Sum2 : Sum  Inputs=-+
  Unit Delay{1..7} (7 alike) : UnitDelay  SampleTime=-1  HasFrameUpgradeWarning=on
  Voltage Slew : RateLimiter  RisingSlewLimit=VslewDC  FallingSlewLimit=-VslewDC  SampleTimeMode=inherited  LinearizeAsGain=off
  Vin : Outport  VectorParamsAs1DForOutWhenUnconnected=off
  wires:
  Memory/1 -> MATLAB Function/4(x)
  Sum2/1 -> MATLAB Function/2(v)
  Sum1/1 -> MATLAB Function/3(i)
  Sum/1 -> MATLAB Function/1(p)
  Pout/1 -> Unit Delay2/1
  Iout/1 -> Unit Delay3/1
  MATLAB Function/1(y) -> Unit Delay4/1
  P_set/1 -> Power Slew/1
  V_set/1 -> Voltage Slew/1
  I_set/1 -> Current Slew/1
  Current Slew/1 -> Unit Delay7/1
  Voltage Slew/1 -> Unit Delay6/1
  Power Slew/1 -> Unit Delay5/1
  Unit Delay2/1 -> Sum/1
  Vout/1 -> Unit Delay1/1
  Unit Delay3/1 -> Sum1/1
  Unit Delay4/1 -> Vin/1, Memory/1
  Unit Delay1/1 -> Sum2/1
  Unit Delay5/1 -> Sum/2
  Unit Delay6/1 -> Sum2/2
  Unit Delay7/1 -> Sum1/2

== system NHR9410Model24k_2020b/NHR 9410/Chanel-3/Chanel-3 Control/All DC (mode-4) control1 ==
  Pout : Inport
  Vout : Inport  Port=2
  Iout : Inport  Port=3
  P_set : Inport  Port=4
  V_set : Inport  Port=5
  I_set : Inport  Port=6
  Enable : EnablePort
  Current Slew : RateLimiter  RisingSlewLimit=IslewDC  FallingSlewLimit=-IslewDC  SampleTimeMode=inherited  LinearizeAsGain=off
  MATLAB Function : MATLAB Function  TreatAsAtomicUnit=on
  Memory : Memory
  Power Slew : RateLimiter  RisingSlewLimit=PslewDC  FallingSlewLimit=-PslewDC  SampleTimeMode=inherited  LinearizeAsGain=off
  Scope : Scope
  Sum : Sum  Inputs=-+
  Sum1 : Sum  Inputs=-+
  Sum2 : Sum  Inputs=-+
  Unit Delay{,1..5} (6 alike) : UnitDelay  SampleTime=-1  HasFrameUpgradeWarning=on
  Voltage Slew : RateLimiter  RisingSlewLimit=VslewDC  FallingSlewLimit=-VslewDC  SampleTimeMode=inherited  LinearizeAsGain=off
  Vin : Outport  VectorParamsAs1DForOutWhenUnconnected=off
  wires:
  Memory/1 -> MATLAB Function/4(x)
  Sum2/1 -> MATLAB Function/2(v)
  Sum1/1 -> MATLAB Function/3(i)
  Sum/1 -> MATLAB Function/1(p)
  MATLAB Function/1(y) -> Scope/1, Vin/1, Memory/1
  P_set/1 -> Power Slew/1
  V_set/1 -> Voltage Slew/1
  I_set/1 -> Current Slew/1
  Current Slew/1 -> Unit Delay2/1
  Voltage Slew/1 -> Unit Delay1/1
  Power Slew/1 -> Unit Delay3/1
  Pout/1 -> Unit Delay5/1
  Iout/1 -> Unit Delay4/1
  Vout/1 -> Unit Delay/1
  Unit Delay3/1 -> Sum/2
  Unit Delay1/1 -> Sum2/2
  Unit Delay2/1 -> Sum1/2
  Unit Delay4/1 -> Sum1/1
  Unit Delay/1 -> Sum2/1
  Unit Delay5/1 -> Sum/1

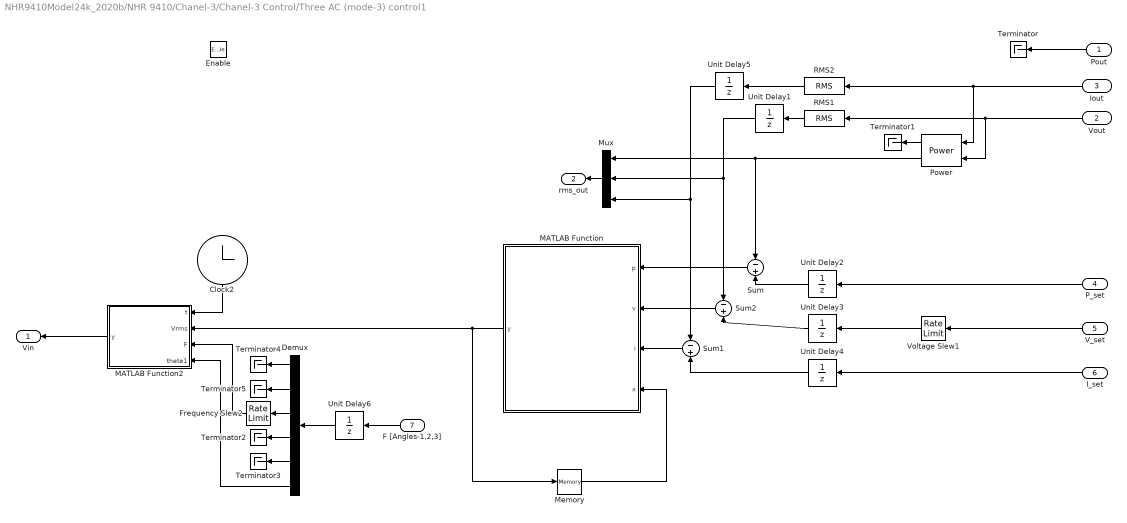
== system NHR9410Model24k_2020b/NHR 9410/Chanel-3/Chanel-3 Control/Three AC (mode-3) control1 ==
  Pout : Inport
  Vout : Inport  Port=2
  Iout : Inport  Port=3
  P_set : Inport  Port=4
  V_set : Inport  Port=5
  I_set : Inport  Port=6
  F [Angles-1,2,3] : Inport  Port=7
  Enable : EnablePort
  Clock2 : Clock
  Demux : Demux  Outputs=6
  Frequency Slew2 : RateLimiter  RisingSlewLimit=FslewAC  FallingSlewLimit=-FslewAC  SampleTimeMode=inherited  LinearizeAsGain=off
  MATLAB Function : MATLAB Function  TreatAsAtomicUnit=on
  MATLAB Function2 : MATLAB Function  TreatAsAtomicUnit=on
  Memory : Memory
  Mux : Mux  Inputs=3
  Power : powerlib_meascontrol/Measurements/Power  Freq=60  Vinit=[0, 0]  Iinit=[0, 0]  Ts=0
  RMS1 : powerlib_meascontrol/Measurements/RMS  TrueRMS=on  Freq=60  RMSInit=0  Ts=0
  RMS2 : powerlib_meascontrol/Measurements/RMS  TrueRMS=on  Freq=60  RMSInit=0  Ts=0
  Sum : Sum  Inputs=-+
  Sum1 : Sum  Inputs=-+
  Sum2 : Sum  Inputs=-+
  Terminator{,1..5} (6 alike) : Terminator
  Unit Delay{1..6} (6 alike) : UnitDelay  SampleTime=-1  HasFrameUpgradeWarning=on
  Voltage Slew1 : RateLimiter  RisingSlewLimit=VslewAC  FallingSlewLimit=-VslewAC  SampleTimeMode=inherited  LinearizeAsGain=off
  Vin : Outport  VectorParamsAs1DForOutWhenUnconnected=off
  rms_out : Outport  Port=2  VectorParamsAs1DForOutWhenUnconnected=off
  wires:
  Vout/1 -> RMS1/1, Power/1
  MATLAB Function/1(y) -> MATLAB Function2/2(Vrms), Memory/1
  Iout/1 -> RMS2/1, Power/2
  Pout/1 -> Terminator/1
  Power/2 -> Terminator1/1
  Sum/1 -> MATLAB Function/1(p)
  Sum2/1 -> MATLAB Function/2(v)
  Sum1/1 -> MATLAB Function/3(i)
  I_set/1 -> Unit Delay4/1
  P_set/1 -> Unit Delay2/1
  RMS1/1 -> Unit Delay1/1
  RMS2/1 -> Unit Delay5/1
  Memory/1 -> MATLAB Function/4(x)
  Clock2/1 -> MATLAB Function2/1(t)
  MATLAB Function2/1(y) -> Vin/1
  Power/1 -> Sum/1, Mux/1
  Mux/1 -> rms_out/1
  F [Angles-1,2,3]/1 -> Unit Delay6/1
  Demux/1 -> Terminator4/1
  Demux/4 -> Terminator2/1
  V_set/1 -> Voltage Slew1/1
  Demux/2 -> Terminator5/1
  Demux/5 -> Terminator3/1
  Demux/3 -> Frequency Slew2/1
  Demux/6 -> MATLAB Function2/4(theta1)
  Frequency Slew2/1 -> MATLAB Function2/3(F)
  Voltage Slew1/1 -> Unit Delay3/1
  Unit Delay5/1 -> Sum1/1, Mux/3
  Unit Delay1/1 -> Sum2/1, Mux/2
  Unit Delay2/1 -> Sum/2
  Unit Delay3/1 -> Sum2/2
  Unit Delay4/1 -> Sum1/2
  Unit Delay6/1 -> Demux/1

== system NHR9410Model24k_2020b/NHR 9410 Safety Settings/Safety Ch-1/Trip signal generator (max) Sink Current/trip signal gen ==
  signal in : Inport
  Enable : EnablePort
  -1 : Constant  OutDataTypeStr=boolean
  -2 : Constant  OutDataTypeStr=boolean
  -3 : Constant  OutDataTypeStr=boolean
  -4 : Constant  Value=0  OutDataTypeStr=boolean
  -5 : Constant  Value=0  OutDataTypeStr=boolean
  -7 : Constant  Value=trip_t  OutDataTypeStr=boolean
  Add : Sum
  Compare To Constant : simulink/Logic and Bit Operations/Compare To Constant  relop=>  const=0  OutDataTypeStr=uint8
  Compare To Constant1 : simulink/Logic and Bit Operations/Compare To Constant  relop===  const=0  OutDataTypeStr=uint8
  D Latch1 : simulink_extras/Flip Flops/D Latch
      settings: SourceProductBaseCode=SL
  Data Type Conversion : DataTypeConversion  OutDataTypeStr=double
  Data Type Conversion1 : DataTypeConversion  OutDataTypeStr=double
  Gain : Gain  Gain=2
  Gain1 : Gain
  Logical Operator1 : Logic  AllPortsSameDT=off  OutDataTypeStr=boolean
  Multiport Switch : MultiPortSwitch  Inputs=2  DataPortForDefault=Additional data port
  On Delay : powerlib_meascontrol/Logic/On Delay  DelayType=On delay  delay=trip_t  ic=0  Ts=0
  Switch : Switch  Criteria=u2 > Threshold  Threshold=trip_thres
  Terminator1 : Terminator
  trip_out : Outport  VectorParamsAs1DForOutWhenUnconnected=off
  wires:
  Switch/1 -> On Delay/1, Logical Operator1/2
  On Delay/1 -> D Latch1/2
  D Latch1/1 -> Multiport Switch/2
  -4/1 -> Multiport Switch/4
  Multiport Switch/1 -> trip_out/1
  -2/1 -> Multiport Switch/3
  -3/1 -> Switch/1
  -5/1 -> Switch/3
  Logical Operator1/1 -> D Latch1/1
  D Latch1/2 -> Terminator1/1
  signal in/1 -> Switch/2
  -1/1 -> Logical Operator1/1
  -7/1 -> Compare To Constant1/1, Compare To Constant/1
  Gain1/1 -> Add/1
  Data Type Conversion/1 -> Gain1/1
  Gain/1 -> Add/2
  Data Type Conversion1/1 -> Gain/1
  Compare To Constant1/1 -> Data Type Conversion1/1
  Compare To Constant/1 -> Data Type Conversion/1
  Add/1 -> Multiport Switch/1

== system NHR9410Model24k_2020b/NHR 9410 Safety Settings/Safety Ch-1/Trip signal generator (max) Sink Power/trip signal gen ==
  signal in : Inport
  Enable : EnablePort
  -1 : Constant  OutDataTypeStr=boolean
  -2 : Constant  OutDataTypeStr=boolean
  -3 : Constant  OutDataTypeStr=boolean
  -4 : Constant  Value=0  OutDataTypeStr=boolean
  -5 : Constant  Value=0  OutDataTypeStr=boolean
  -7 : Constant  Value=trip_t  OutDataTypeStr=boolean
  Add : Sum
  Compare To Constant : simulink/Logic and Bit Operations/Compare To Constant  relop=>  const=0  OutDataTypeStr=uint8
  Compare To Constant1 : simulink/Logic and Bit Operations/Compare To Constant  relop===  const=0  OutDataTypeStr=uint8
  D Latch1 : simulink_extras/Flip Flops/D Latch
      settings: SourceProductBaseCode=SL
  Data Type Conversion : DataTypeConversion  OutDataTypeStr=double
  Data Type Conversion1 : DataTypeConversion  OutDataTypeStr=double
  Gain : Gain  Gain=2
  Gain1 : Gain
  Logical Operator1 : Logic  AllPortsSameDT=off  OutDataTypeStr=boolean
  Multiport Switch : MultiPortSwitch  Inputs=2  DataPortForDefault=Additional data port
  On Delay : powerlib_meascontrol/Logic/On Delay  DelayType=On delay  delay=trip_t  ic=0  Ts=0
  Switch : Switch  Criteria=u2 > Threshold  Threshold=trip_thres
  Terminator1 : Terminator
  trip_out : Outport  VectorParamsAs1DForOutWhenUnconnected=off
  wires:
  -1/1 -> Logical Operator1/1
  signal in/1 -> Switch/2
  D Latch1/2 -> Terminator1/1
  Logical Operator1/1 -> D Latch1/1
  -5/1 -> Switch/3
  -3/1 -> Switch/1
  -2/1 -> Multiport Switch/3
  Multiport Switch/1 -> trip_out/1
  -4/1 -> Multiport Switch/4
  D Latch1/1 -> Multiport Switch/2
  On Delay/1 -> D Latch1/2
  Switch/1 -> Logical Operator1/2, On Delay/1
  -7/1 -> Compare To Constant1/1, Compare To Constant/1
  Gain1/1 -> Add/1
  Data Type Conversion/1 -> Gain1/1
  Gain/1 -> Add/2
  Data Type Conversion1/1 -> Gain/1
  Compare To Constant1/1 -> Data Type Conversion1/1
  Compare To Constant/1 -> Data Type Conversion/1
  Add/1 -> Multiport Switch/1

== system NHR9410Model24k_2020b/NHR 9410 Safety Settings/Safety Ch-1/Trip signal generator (max) Source Current/trip signal gen ==
  signal in : Inport
  Enable : EnablePort
  -1 : Constant  OutDataTypeStr=boolean
  -2 : Constant  OutDataTypeStr=boolean
  -3 : Constant  OutDataTypeStr=boolean
  -4 : Constant  Value=0  OutDataTypeStr=boolean
  -5 : Constant  Value=0  OutDataTypeStr=boolean
  -7 : Constant  Value=trip_t  OutDataTypeStr=boolean
  Add : Sum
  Compare To Constant : simulink/Logic and Bit Operations/Compare To Constant  relop=>  const=0  OutDataTypeStr=uint8
  Compare To Constant1 : simulink/Logic and Bit Operations/Compare To Constant  relop===  const=0  OutDataTypeStr=uint8
  D Latch1 : simulink_extras/Flip Flops/D Latch
      settings: SourceProductBaseCode=SL
  Data Type Conversion : DataTypeConversion  OutDataTypeStr=double
  Data Type Conversion1 : DataTypeConversion  OutDataTypeStr=double
  Gain : Gain  Gain=2
  Gain1 : Gain
  Logical Operator1 : Logic  AllPortsSameDT=off  OutDataTypeStr=boolean
  Multiport Switch : MultiPortSwitch  Inputs=2  DataPortForDefault=Additional data port
  On Delay : powerlib_meascontrol/Logic/On Delay  DelayType=On delay  delay=trip_t  ic=0  Ts=0
  Switch : Switch  Criteria=u2 > Threshold  Threshold=trip_thres
  Terminator1 : Terminator
  trip_out : Outport  VectorParamsAs1DForOutWhenUnconnected=off
  wires:
  -1/1 -> Logical Operator1/1
  signal in/1 -> Switch/2
  D Latch1/2 -> Terminator1/1
  Logical Operator1/1 -> D Latch1/1
  -5/1 -> Switch/3
  -3/1 -> Switch/1
  -2/1 -> Multiport Switch/3
  Multiport Switch/1 -> trip_out/1
  -4/1 -> Multiport Switch/4
  D Latch1/1 -> Multiport Switch/2
  On Delay/1 -> D Latch1/2
  Switch/1 -> Logical Operator1/2, On Delay/1
  -7/1 -> Compare To Constant1/1, Compare To Constant/1
  Gain1/1 -> Add/1
  Data Type Conversion/1 -> Gain1/1
  Add/1 -> Multiport Switch/1
  Gain/1 -> Add/2
  Data Type Conversion1/1 -> Gain/1
  Compare To Constant1/1 -> Data Type Conversion1/1
  Compare To Constant/1 -> Data Type Conversion/1

== system NHR9410Model24k_2020b/NHR 9410 Safety Settings/Safety Ch-1/Trip signal generator (max) Source Power/trip signal gen ==
  signal in : Inport
  Enable : EnablePort
  -1 : Constant  OutDataTypeStr=boolean
  -2 : Constant  OutDataTypeStr=boolean
  -3 : Constant  OutDataTypeStr=boolean
  -4 : Constant  Value=0  OutDataTypeStr=boolean
  -5 : Constant  Value=0  OutDataTypeStr=boolean
  -7 : Constant  Value=trip_t  OutDataTypeStr=boolean
  Add : Sum
  Compare To Constant : simulink/Logic and Bit Operations/Compare To Constant  relop=>  const=0  OutDataTypeStr=uint8
  Compare To Constant1 : simulink/Logic and Bit Operations/Compare To Constant  relop===  const=0  OutDataTypeStr=uint8
  D Latch1 : simulink_extras/Flip Flops/D Latch
      settings: SourceProductBaseCode=SL
  Data Type Conversion : DataTypeConversion  OutDataTypeStr=double
  Data Type Conversion1 : DataTypeConversion  OutDataTypeStr=double
  Gain : Gain  Gain=2
  Gain1 : Gain
  Logical Operator1 : Logic  AllPortsSameDT=off  OutDataTypeStr=boolean
  Multiport Switch : MultiPortSwitch  Inputs=2  DataPortForDefault=Additional data port
  On Delay : powerlib_meascontrol/Logic/On Delay  DelayType=On delay  delay=trip_t  ic=0  Ts=0
  Switch : Switch  Criteria=u2 > Threshold  Threshold=trip_thres
  Terminator1 : Terminator
  trip_out : Outport  VectorParamsAs1DForOutWhenUnconnected=off
  wires:
  Switch/1 -> On Delay/1, Logical Operator1/2
  On Delay/1 -> D Latch1/2
  D Latch1/1 -> Multiport Switch/2
  -4/1 -> Multiport Switch/4
  Multiport Switch/1 -> trip_out/1
  -2/1 -> Multiport Switch/3
  -3/1 -> Switch/1
  -5/1 -> Switch/3
  Logical Operator1/1 -> D Latch1/1
  D Latch1/2 -> Terminator1/1
  signal in/1 -> Switch/2
  -1/1 -> Logical Operator1/1
  -7/1 -> Compare To Constant1/1, Compare To Constant/1
  Gain1/1 -> Add/1
  Data Type Conversion/1 -> Gain1/1
  Gain/1 -> Add/2
  Data Type Conversion1/1 -> Gain/1
  Compare To Constant1/1 -> Data Type Conversion1/1
  Compare To Constant/1 -> Data Type Conversion/1
  Add/1 -> Multiport Switch/1

== system NHR9410Model24k_2020b/NHR 9410 Safety Settings/Safety Ch-1/Trip signal generator (max) Voltage/trip signal gen ==
  signal in : Inport
  Enable : EnablePort
  -1 : Constant  OutDataTypeStr=boolean
  -2 : Constant  OutDataTypeStr=boolean
  -3 : Constant  OutDataTypeStr=boolean
  -4 : Constant  Value=0  OutDataTypeStr=boolean
  -5 : Constant  Value=0  OutDataTypeStr=boolean
  -7 : Constant  Value=trip_t  OutDataTypeStr=boolean
  Add : Sum
  Compare To Constant : simulink/Logic and Bit Operations/Compare To Constant  relop=>  const=0  OutDataTypeStr=uint8
  Compare To Constant1 : simulink/Logic and Bit Operations/Compare To Constant  relop===  const=0  OutDataTypeStr=uint8
  D Latch1 : simulink_extras/Flip Flops/D Latch
      settings: SourceProductBaseCode=SL
  Data Type Conversion : DataTypeConversion  OutDataTypeStr=double
  Data Type Conversion1 : DataTypeConversion  OutDataTypeStr=double
  Gain : Gain  Gain=2
  Gain1 : Gain
  Logical Operator1 : Logic  AllPortsSameDT=off  OutDataTypeStr=boolean
  Multiport Switch : MultiPortSwitch  Inputs=2  DataPortForDefault=Additional data port
  On Delay : powerlib_meascontrol/Logic/On Delay  DelayType=On delay  delay=trip_t  ic=0  Ts=0
  Switch : Switch  Criteria=u2 > Threshold  Threshold=trip_thres
  Terminator1 : Terminator
  trip_out : Outport  VectorParamsAs1DForOutWhenUnconnected=off
  wires:
  Switch/1 -> On Delay/1, Logical Operator1/2
  On Delay/1 -> D Latch1/2
  D Latch1/1 -> Multiport Switch/2
  -4/1 -> Multiport Switch/4
  Multiport Switch/1 -> trip_out/1
  -2/1 -> Multiport Switch/3
  -3/1 -> Switch/1
  -5/1 -> Switch/3
  Logical Operator1/1 -> D Latch1/1
  D Latch1/2 -> Terminator1/1
  signal in/1 -> Switch/2
  -1/1 -> Logical Operator1/1
  -7/1 -> Compare To Constant1/1, Compare To Constant/1
  Gain1/1 -> Add/1
  Gain/1 -> Add/2
  Data Type Conversion1/1 -> Gain/1
  Compare To Constant1/1 -> Data Type Conversion1/1
  Add/1 -> Multiport Switch/1
  Data Type Conversion/1 -> Gain1/1
  Compare To Constant/1 -> Data Type Conversion/1

== system NHR9410Model24k_2020b/NHR 9410 Safety Settings/Safety Ch-1/Trip signal generator (min) Voltage/trip signal gen ==
  signal in : Inport
  Enable : EnablePort
  -1 : Constant  OutDataTypeStr=boolean
  -2 : Constant  OutDataTypeStr=boolean
  -3 : Constant  Value=0  OutDataTypeStr=boolean
  -4 : Constant  Value=0  OutDataTypeStr=boolean
  -5 : Constant  OutDataTypeStr=boolean
  -7 : Constant  Value=trip_t  OutDataTypeStr=boolean
  Add : Sum
  Compare To Constant : simulink/Logic and Bit Operations/Compare To Constant  relop=>  const=0  OutDataTypeStr=uint8
  Compare To Constant1 : simulink/Logic and Bit Operations/Compare To Constant  relop===  const=0  OutDataTypeStr=uint8
  D Latch1 : simulink_extras/Flip Flops/D Latch
      settings: SourceProductBaseCode=SL
  Data Type Conversion : DataTypeConversion  OutDataTypeStr=double
  Data Type Conversion1 : DataTypeConversion  OutDataTypeStr=double
  Gain : Gain  Gain=2
  Gain1 : Gain
  Logical Operator1 : Logic  AllPortsSameDT=off  OutDataTypeStr=boolean
  Multiport Switch : MultiPortSwitch  Inputs=2  DataPortForDefault=Additional data port
  On Delay : powerlib_meascontrol/Logic/On Delay  DelayType=On delay  delay=trip_t  ic=0  Ts=0
  Switch : Switch  Criteria=u2 > Threshold  Threshold=trip_thres
  Terminator1 : Terminator
  trip_out : Outport  VectorParamsAs1DForOutWhenUnconnected=off
  wires:
  -1/1 -> Logical Operator1/1
  signal in/1 -> Switch/2
  D Latch1/2 -> Terminator1/1
  Logical Operator1/1 -> D Latch1/1
  -5/1 -> Switch/3
  -3/1 -> Switch/1
  -2/1 -> Multiport Switch/3
  Multiport Switch/1 -> trip_out/1
  -4/1 -> Multiport Switch/4
  D Latch1/1 -> Multiport Switch/2
  On Delay/1 -> D Latch1/2
  Switch/1 -> Logical Operator1/2, On Delay/1
  Gain1/1 -> Add/1
  Compare To Constant/1 -> Data Type Conversion/1
  Gain/1 -> Add/2
  Compare To Constant1/1 -> Data Type Conversion1/1
  Data Type Conversion1/1 -> Gain/1
  -7/1 -> Compare To Constant1/1, Compare To Constant/1
  Data Type Conversion/1 -> Gain1/1
  Add/1 -> Multiport Switch/1

== system NHR9410Model24k_2020b/NHR 9410 Safety Settings/Safety Ch-1/Trip signal generator (peak) Current/trip signal gen ==
  signal in : Inport
  Enable : EnablePort
  -2 : Constant  OutDataTypeStr=boolean
  -4 : Constant  Value=0  OutDataTypeStr=boolean
  D Latch1 : simulink_extras/Flip Flops/D Latch
      settings: SourceProductBaseCode=SL
  Data Type Conversion : DataTypeConversion  OutDataTypeStr=boolean
  Switch1 : Switch  Criteria=u2 > Threshold  Threshold=trip_thres
  Terminator1 : Terminator
  trip_out : Outport  VectorParamsAs1DForOutWhenUnconnected=off
  wires:
  -4/1 -> Switch1/3
  Switch1/1 -> D Latch1/2, Data Type Conversion/1
  D Latch1/1 -> trip_out/1
  D Latch1/2 -> Terminator1/1
  -2/1 -> Switch1/1
  Data Type Conversion/1 -> D Latch1/1
  signal in/1 -> Switch1/2

== system NHR9410Model24k_2020b/NHR 9410 Safety Settings/Safety Ch-1/Trip signal generator (peak) Voltage/trip signal gen ==
  signal in : Inport
  Enable : EnablePort
  -2 : Constant  OutDataTypeStr=boolean
  -4 : Constant  Value=0  OutDataTypeStr=boolean
  D Latch1 : simulink_extras/Flip Flops/D Latch
      settings: SourceProductBaseCode=SL
  Data Type Conversion : DataTypeConversion  OutDataTypeStr=boolean
  Switch1 : Switch  Criteria=u2 > Threshold  Threshold=trip_thres
  Terminator1 : Terminator
  trip_out : Outport  VectorParamsAs1DForOutWhenUnconnected=off
  wires:
  signal in/1 -> Switch1/2
  Data Type Conversion/1 -> D Latch1/1
  -2/1 -> Switch1/1
  D Latch1/2 -> Terminator1/1
  Switch1/1 -> D Latch1/2, Data Type Conversion/1
  -4/1 -> Switch1/3
  D Latch1/1 -> trip_out/1

== system NHR9410Model24k_2020b/NHR 9410 Safety Settings/Safety Ch-2/Trip signal generator (max) Sink Current/trip signal gen ==
  signal in : Inport
  Enable : EnablePort
  -1 : Constant  OutDataTypeStr=boolean
  -2 : Constant  OutDataTypeStr=boolean
  -3 : Constant  OutDataTypeStr=boolean
  -4 : Constant  Value=0  OutDataTypeStr=boolean
  -5 : Constant  Value=0  OutDataTypeStr=boolean
  -7 : Constant  Value=trip_t  OutDataTypeStr=boolean
  Add : Sum
  Compare To Constant : simulink/Logic and Bit Operations/Compare To Constant  relop=>  const=0  OutDataTypeStr=uint8
  Compare To Constant1 : simulink/Logic and Bit Operations/Compare To Constant  relop===  const=0  OutDataTypeStr=uint8
  D Latch1 : simulink_extras/Flip Flops/D Latch
      settings: SourceProductBaseCode=SL
  Data Type Conversion : DataTypeConversion  OutDataTypeStr=double
  Data Type Conversion1 : DataTypeConversion  OutDataTypeStr=double
  Gain : Gain  Gain=2
  Gain1 : Gain
  Logical Operator1 : Logic  AllPortsSameDT=off  OutDataTypeStr=boolean
  Multiport Switch : MultiPortSwitch  Inputs=2  DataPortForDefault=Additional data port
  On Delay : powerlib_meascontrol/Logic/On Delay  DelayType=On delay  delay=trip_t  ic=0  Ts=0
  Switch : Switch  Criteria=u2 > Threshold  Threshold=trip_thres
  Terminator1 : Terminator
  trip_out : Outport  VectorParamsAs1DForOutWhenUnconnected=off
  wires:
  -1/1 -> Logical Operator1/1
  signal in/1 -> Switch/2
  D Latch1/2 -> Terminator1/1
  Logical Operator1/1 -> D Latch1/1
  -5/1 -> Switch/3
  -3/1 -> Switch/1
  -2/1 -> Multiport Switch/3
  Multiport Switch/1 -> trip_out/1
  -4/1 -> Multiport Switch/4
  D Latch1/1 -> Multiport Switch/2
  On Delay/1 -> D Latch1/2
  Switch/1 -> Logical Operator1/2, On Delay/1
  -7/1 -> Compare To Constant1/1, Compare To Constant/1
  Gain1/1 -> Add/1
  Data Type Conversion/1 -> Gain1/1
  Add/1 -> Multiport Switch/1
  Gain/1 -> Add/2
  Data Type Conversion1/1 -> Gain/1
  Compare To Constant1/1 -> Data Type Conversion1/1
  Compare To Constant/1 -> Data Type Conversion/1
